simulink model "controla_planta_ROS"  (R2025b)
settings: Solver=ode14x  StartTime=0.0  StopTime=20  FixedStep=0.01  RelTol=1e-3
InitFcn:
  | start_time_epoch = posixtime(datetime('now'))-3600;
  | setenv('ROS_LOCALHOST_ONLY', '');
  | setenv('RMW_IMPLEMENTATION','rmw_cyclonedds_cpp')
values from neighbouring files (symbols this model uses):
  cc = 4.08    [parametros_planta.m]
  cp = 0.0002    [parametros_planta.m]
  g = 9.81    [parametros_planta.m]
  J = 0.0139    [parametros_planta.m]
  lcm = 0.3    [parametros_planta.m]
  M = mp + mc    (= 1.2)    [parametros_planta.m]
  mc = 1.08    [parametros_planta.m]
  mp = 0.12    [parametros_planta.m]
undefined symbols (not defined in the file or in its folder): K_lqr
libraries: ros2lib x2
settings Model: Creator=miguel  LastModifiedBy=miguel
settings SolverCC: EnableFixedStepZeroCrossing=on
settings OptimizationCC: DefaultParameterBehavior=Inlined  EnhancedBackFolding=on  PassReuseOutputArgsAs=Individual arguments  ZeroExternalMemoryAtStartup=off  ZeroInternalMemoryAtStartup=off  MaxStackSize=64  OptimizeBlockOrder=speed  DifferentSizesBufferReuse=on  OptimizationCustomize=off  EfficientTunableParamExpr=on
settings DebuggingCC: ParameterTunabilityLossMsg=error
settings HardwareCC: ProdBitPerLong=64.0  ProdHWDeviceType=Intel->x86-64 (Linux 64)  UseEmbeddedCoderFeatures=off
settings SFSimCC: MATLABDynamicMemAlloc=off
settings RTWCC: SystemTargetFile=ert.tlc  HardwareBoard=Robot Operating System 2 (ROS 2)  TLCOptions="-aInlineSetEventsForThisBaseRateFcn=TLC_FALSE -aSuppressMultiTaskScheduler=TLC_FALSE  -aRateBasedStepFcn=0"  TemplateMakefile=ert_default_tmf  Toolchain=Colcon Tools  TargetLang=C++  Description=Embedded Coder
settings CodeAppCC: ForceParamTrailComments=on  IgnoreCustomStorageClasses=off  OperatorAnnotations=on  SimulinkDataObjDesc=on  SFDataObjDesc=on  InsertBlockDesc=on
settings ERTTargetCC: ExtModeTransport=2.0  ExtModeStaticAlloc=on  ExtModeAutomaticAllocSize=off  ExtModeMexFile=ext_xcp  ExtModeIntrfLevel=Level2 - Open  RootIOFormat=Structure reference  CodeInterfacePackaging=C++ class  SupportNonInlinedSFcns=on

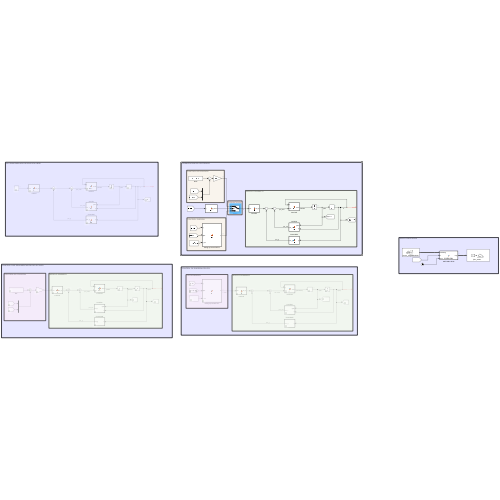
[thumbnail: Simulink's stored preview of the top-level diagram]
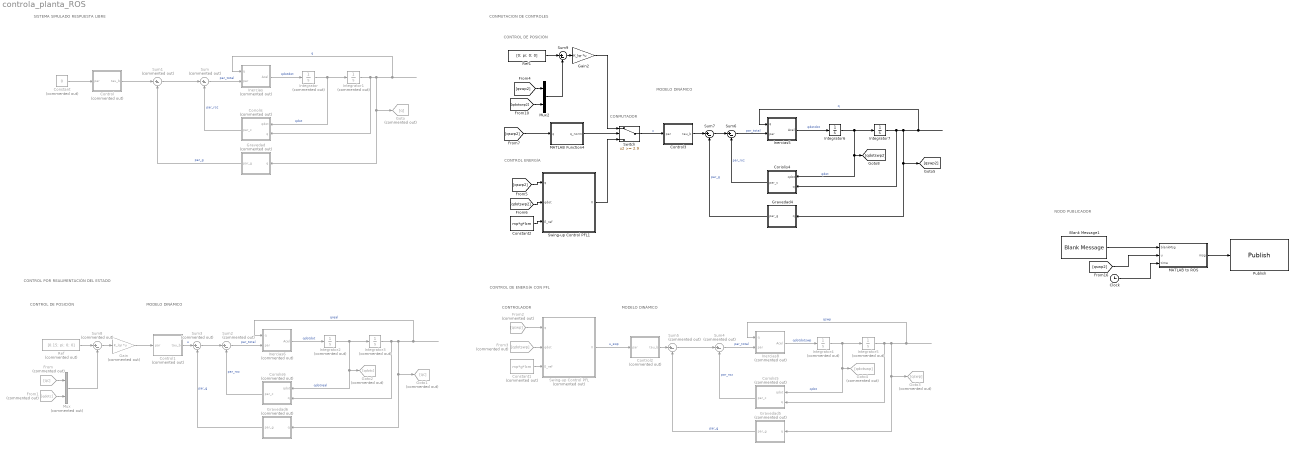
== system controla_planta_ROS ==
  note: CONTROLADOR
  note: MODELO DINÁMICO
  note: CONTROL DE POSICIÓN
  note: MODELO DINÁMICO
  note: CONMUTADOR
  note: MODELO DINÁMICO
  note: CONTROL ENERGÍA
  note: CONTROL DE POSICIÓN
  note: SISTEMA SIMULADO RESPUESTA LIBRE
  note: NODO PUBLICADOR
  note: CONTROL POR REALIMENTACIÓN DEL ESTADO
  note: CONTROL DE ENERGÍA CON PFL
  note: CONMUTACION DE CONTROLES
  Blank Message1 : ros2lib/Blank Message  messageClass=Message  entityType=sensor_msgs/JointState  messageType=sensor_msgs/JointState  SampleTime=inf
  Clock : Clock
  Constant : Constant  Commented=on  Value=0
  Constant1 : Constant  Commented=on  Value=mp*g*lcm
  Constant2 : Constant  Value=mp*g*lcm
  Control : MATLAB Function  Commented=on  TreatAsAtomicUnit=on
  Control1 : MATLAB Function  Commented=on  TreatAsAtomicUnit=on
  Control2 : MATLAB Function  Commented=on  TreatAsAtomicUnit=on
  Control3 : MATLAB Function  TreatAsAtomicUnit=on
  Coriolis : MATLAB Function  Commented=on  TreatAsAtomicUnit=on
  Coriolis4 : MATLAB Function  TreatAsAtomicUnit=on
  Coriolis5 : MATLAB Function  Commented=on  TreatAsAtomicUnit=on
  Coriolis6 : MATLAB Function  Commented=on  TreatAsAtomicUnit=on
  From : From  Commented=on  GotoTag=qc
  From1 : From  Commented=on  GotoTag=qdotc
  From2 : From  Commented=on  GotoTag=qswp
  From3 : From  Commented=on  GotoTag=qdotswp
  Gain : Gain  Commented=on  Gain=K_lqr  Multiplication=Matrix(K*u)
  Gain2 : Gain  Gain=K_lqr  Multiplication=Matrix(K*u)
  Goto : Goto  Commented=on  GotoTag=q
  Goto1 : Goto  Commented=on  GotoTag=qc
  Goto2 : Goto  Commented=on  GotoTag=qdotc
  Goto3 : Goto  Commented=on  GotoTag=qswp
  Goto4 : Goto  Commented=on  GotoTag=qdotswp
  Gravedad : MATLAB Function  Commented=on  TreatAsAtomicUnit=on
  Gravedad4 : MATLAB Function  TreatAsAtomicUnit=on
  Gravedad5 : MATLAB Function  Commented=on  TreatAsAtomicUnit=on
  Gravedad6 : MATLAB Function  Commented=on  TreatAsAtomicUnit=on
  Inercias : MATLAB Function  Commented=on  TreatAsAtomicUnit=on
  Inercias5 : MATLAB Function  TreatAsAtomicUnit=on
  Inercias6 : MATLAB Function  Commented=on  TreatAsAtomicUnit=on
  Inercias8 : MATLAB Function  Commented=on  TreatAsAtomicUnit=on
  Integrator : Integrator  Commented=on  InitialCondition=[0; 0]
  Integrator1 : Integrator  Commented=on  InitialCondition=[0; 3.14]
  Integrator2 : Integrator  Commented=on  InitialCondition=[0; 0]
  Integrator3 : Integrator  Commented=on  InitialCondition=[0; 3.20]
  Integrator4 : Integrator  Commented=on  InitialCondition=[0; 0.01]
  Integrator5 : Integrator  Commented=on  InitialCondition=[0; 0]
  Integrator6 : Integrator  InitialCondition=[0; 0.01]
  Integrator7 : Integrator  InitialCondition=[0; 0]
  MATLAB Function4 : MATLAB Function  TreatAsAtomicUnit=on
  MATLAB to ROS : MATLAB Function  TreatAsAtomicUnit=on
  Mux : Mux  Commented=on  Inputs=2
  Mux2 : Mux  Inputs=2
  Publish : ros2lib/Publish  topicSource=Specify your own  topic=/joint_states  messageType=sensor_msgs/JointState  QOSHistory=Keep last  QOSDepth=10  QOSReliability=Reliable  QOSDurability=Volatile  QOSDeadline=Inf  QOSLifespan=Inf  QOSLiveliness=Automatic  QOSLeaseDuration=Inf  QOSAvoidROSNamespaceConventions=off
  Ref : Constant  Commented=on  Value=[0.15; pi; 0; 0]
  Ref1 : Constant  Value=[0; pi; 0; 0]
  Sum{,1..5,8} (7 alike) : Sum  Commented=on  Inputs=|+-
  Sum6 : Sum  Inputs=|+-
  Sum7 : Sum  Inputs=|+-
  Sum9 : Sum  Inputs=|+-
  Swing-up Control PFL : MATLAB Function  Commented=on  TreatAsAtomicUnit=on
  Swing-up Control PFL1 : MATLAB Function  TreatAsAtomicUnit=on
  Switch : Switch  Threshold=2.9  SaturateOnIntegerOverflow=off  InputSameDT=off
  wires:
  Sum1/1 -> Sum/1
  Gravedad/1(par_g) -> Sum1/2  "par_g"
  Control/1(tau_b) -> Sum1/1
  Integrator1/1 -> Coriolis/2(q), Goto/1, Gravedad/1(q), Inercias/1(q)  "q"
  Inercias/1(Acel) -> Integrator/1  "qdotdot"
  Constant/1 -> Control/1(par)
  Integrator/1 -> Coriolis/1(qdot), Integrator1/1  "qdot"
  Sum/1 -> Inercias/2(par)  "par_total"
  Coriolis/1(par_c) -> Sum/2  "par_roz"
  Blank Message1/1 -> MATLAB to ROS/1(blankMsg)
  MATLAB to ROS/1(msg) -> Publish/1
  Clock/1 -> MATLAB to ROS/3(time)
  [qswp2] -> MATLAB to ROS/2(u)
  Coriolis6/1(par_c) -> Sum2/2  "par_roz"
  Control1/1(tau_b) -> Sum3/1  "u"
  Integrator3/1 -> Coriolis6/2(q), Gravedad6/1(q), Goto1/1, Inercias6/1(q)  "qreal"
  Inercias6/1(Acel) -> Integrator2/1  "qdotdot"
  Sum2/1 -> Inercias6/2(par)  "par_total"
  Gravedad6/1(par_g) -> Sum3/2  "par_g"
  Sum3/1 -> Sum2/1
  Integrator2/1 -> Coriolis6/1(qdot), Goto2/1, Integrator3/1  "qdotreal"
  From/1 -> Mux/1
  From1/1 -> Mux/2
  Inercias8/1(Acel) -> Integrator4/1  "qdotdotswp"
  Integrator5/1 -> Coriolis5/2(q), Gravedad5/1(q), Goto3/1, Inercias8/1(q)  "qswp"
  Sum5/1 -> Sum4/1
  Gravedad5/1(par_g) -> Sum5/2  "par_g"
  Control2/1(tau_b) -> Sum5/1
  Integrator4/1 -> Coriolis5/1(qdot), Goto4/1, Integrator5/1  "qdot"
  Sum4/1 -> Inercias8/2(par)  "par_total"
  Coriolis5/1(par_c) -> Sum4/2  "par_roz"
  Swing-up Control PFL/1(V) -> Control2/1(par)  "u_swp"
  From2/1 -> Swing-up Control PFL/1(q)
  From3/1 -> Swing-up Control PFL/2(qdot)
  Constant2/1 -> Swing-up Control PFL1/3(E_ref)
  Control3/1(tau_b) -> Sum7/1
  Coriolis4/1(par_c) -> Sum6/2  "par_roz"
  Sum7/1 -> Sum6/1
  Inercias5/1(Acel) -> Integrator6/1  "qdotdot"
  [qdotswp2] -> Swing-up Control PFL1/2(qdot)
  Integrator6/1 -> Coriolis4/1(qdot), [qdotswp2], Integrator7/1  "qdot"
  Sum6/1 -> Inercias5/2(par)  "par_total"
  [qswp2] -> Swing-up Control PFL1/1(q)
  Gravedad4/1(par_g) -> Sum7/2  "par_g"
  Integrator7/1 -> Coriolis4/2(q), Gravedad4/1(q), [qswp2], Inercias5/1(q)  "q"
  Switch/1 -> Control3/1(par)  "u"
  MATLAB Function4/1(q_norm) -> Switch/2
  [qswp2] -> MATLAB Function4/1(q)
  Constant1/1 -> Swing-up Control PFL/3(E_ref)
  Mux/1 -> Sum8/2
  Ref/1 -> Sum8/1
  Gain/1 -> Control1/1(par)
  Sum8/1 -> Gain/1
  Ref1/1 -> Sum9/1
  [qswp2] -> Mux2/1
  Mux2/1 -> Sum9/2
  Sum9/1 -> Gain2/1
  [qdotswp2] -> Mux2/2
  Swing-up Control PFL1/1(V) -> Switch/3
  Gain2/1 -> Switch/1

== matlab function controla_planta_ROS/Control2 ==
  data: par input; tau_b output
function tau_b = B(par)

tau_b = [0.64; 0]*par; %Nuestra acción de control se aplica sobre el eje horizontal.

== matlab function controla_planta_ROS/Gravedad5 ==
  data: q input; par_g output; mp parameter; g parameter; lcm parameter
function par_g = Gq(q, mp, g, lcm)
G = [0; mp*g*lcm*sin(q(2))]; 

par_g = G;

== matlab function controla_planta_ROS/Coriolis5 ==
  data: qdot input; q input; par_c output size=[2, 1]; cc parameter; cp parameter; mp parameter; lcm parameter
function par_c = Cq(qdot, q, cc, cp, mp, lcm)

%Nota: cp = 0 Nm.rad/s no me lo creo habrá que estimarlo de forma
%conservadora.

C = [cc,   -mp*lcm*qdot(2)*sin(q(2))
      0,          cp        ]; 

par_c = C*qdot;

== matlab function controla_planta_ROS/Control3 ==
  data: par input; tau_b output
function tau_b = B(par)

tau_b = [0.64; 0]*par; %Nuestra acción de control se aplica sobre el eje horizontal.

== matlab function controla_planta_ROS/Swing-up Control PFL ==
  data: q input; V output; qdot input; E_ref input; mp parameter; lcm parameter; cp parameter; cc parameter; J parameter; mc parameter
function V = fcn(q, qdot, E_ref, mp, lcm, cp, cc, J, mc) % Añadido Mc y salida F

% --- PARAMETROS FISICOS Y GANANCIAS ---
g = 9.81; % Añadido el punto y coma

% Ganancias del control de energía (Swing-up) AJUSTAR
Ke = 50; 
kp = 8.16; 
kd = 4; 

% -- ESTADOS DEL SISTEMA --
x = q(1);        % Posición del carro
theta = q(2);    % Ángulo del péndulo (0 = arriba)
xdot = qdot(1);  % Velocidad del carro
thetadot = qdot(2); % Velocidad angular

% --- 1. CÁLCULO DE ENERGÍA ---
Ep = -mp * g * lcm * cos(theta); 
Ek = 0.5 * J * thetadot^2;
E_total = Ep + Ek;

% --- 2. LEY DE CONTROL DE ENERGÍA (Aceleración 'u') ---
e = E_total - E_ref;
u = Ke * thetadot * cos(theta) * e - kp * x - kd * xdot;

% --- 3. LINEARIZACIÓN POR RETROALIMENTACIÓN PARCIAL (PFL) ---
% Convierte la aceleración deseada 'u' en Fuerza 'F' para el motor

thetadotdot = 1/J *(-mp*lcm*cos(theta)*u ...
    + mp*g*lcm*sin(theta) -cp*thetadot);

F = (mc + mp) * u ...
    - (mp * lcm * thetadot^2 * sin(theta)) ...
    + (mp * lcm * cos(theta)) * thetadotdot ...
    +cc*xdot;

%Saturacion --> Evitar oscilaciones iniciales bruscas.
F_max = 4; % Newtons
if F > F_max
    F = F_max;
elseif F < -F_max
    F = -F_max;
end

V = F / 0.64;   %Conversión a voltios

end

== matlab function controla_planta_ROS/Gravedad6 ==
  data: q input; par_g output; mp parameter; g parameter; lcm parameter
function par_g = Gq(q, mp, g, lcm)
G = [0; mp*g*lcm*sin(q(2))]; 

par_g = G;

== matlab function controla_planta_ROS/Coriolis6 ==
  data: qdot input; q input; par_c output size=[2, 1]; cc parameter; cp parameter; mp parameter; lcm parameter
function par_c = Cq(qdot, q, cc, cp, mp, lcm)

%Nota: cp = 0 Nm.rad/s no me lo creo habrá que estimarlo de forma
%conservadora.

C = [cc,   -mp*lcm*qdot(2)*sin(q(2))
      0,          cp        ]; 

par_c = C*qdot;

== matlab function controla_planta_ROS/MATLAB Function4 ==
  data: q input; q_norm output
function q_norm = fcn(q)
    % Esto envuelve el ángulo para que siempre esté entre -pi y +pi
    q_norm = atan2(sin(q(2)), cos(q(2)));
    q_norm = abs(q_norm);
end

== matlab function controla_planta_ROS/MATLAB to ROS ==
  data: blankMsg input; msg output Bus: SL_Bus_sensor_msgs_JointState; u input; time input; start_time_epoch parameter
function msg = create_msg(blankMsg, u, time, start_time_epoch)
%#codegen
msg = blankMsg;

%Sincronización con el reloj interno de la máquina.
total_time = start_time_epoch + time; 
%Indicar el tiempo de simulación para que RViz pueda componer la
%simulación. 
s = floor(total_time);
ns = (total_time - s) * 1e9;  
msg.header.stamp.sec = int32(s);
msg.header.stamp.nanosec = uint32(ns);

% Definimos los nombres y sus posiciones correspondientes
strArrayToAssign = {'cart_slider', 'pole_joint'};
% Las posiciones angulares de nuestro péndulo. 
positionsToAssign = [u(1), u(2)]; 

% 1. Configurar NOMBRES (Strings)
numStringsInArray = length(strArrayToAssign);
msg.name_SL_Info.CurrentLength = uint32(numStringsInArray);

for idx=1:numStringsInArray
    str = strArrayToAssign{idx};
    strLength = length(str);
    % Asignar caracteres convertidos a uint8
    msg.name(idx).data(1:strLength) = uint8(str);
    msg.name(idx).data_SL_Info.CurrentLength = uint32(strLength);
end

% 2. Configurar POSICIONES (float64 array)
% El campo 'position' en un Bus de Simulink para JointState 
% también tiene un campo _SL_Info asociado para controlar la longitud.
numPositions = length(positionsToAssign);
msg.position_SL_Info.CurrentLength = uint32(numPositions);
% Asignamos los valores directamente
msg.position(1:numPositions) = positionsToAssign;

% 3. Dejar sin campo de velocidad y esfuerzo el tópico.
msg.velocity_SL_Info.CurrentLength = uint32(0);
msg.effort_SL_Info.CurrentLength = uint32(0);

end

== matlab function controla_planta_ROS/Inercias5 ==
  data: q input; par input; Acel output; J parameter; M parameter; mp parameter; lcm parameter
function Acel = Minv(q,par, J, M, mp, lcm)
%La matriz va aumentando su dimensionalidad a medida que se añaden GDLs

M = [M,          +mp*lcm*cos(q(2));
    +mp*lcm*cos(q(2)),      J]; 

Acel = M\par; %División de matrices.

== matlab function controla_planta_ROS/Coriolis ==
  data: qdot input; q input; par_c output size=[2, 1]; cc parameter; cp parameter; mp parameter; lcm parameter
function par_c = Cq(qdot, q, cc, cp, mp, lcm)

%Nota: cp = 0 Nm.rad/s no me lo creo habrá que estimarlo de forma
%conservadora.

C = [cc,   -mp*lcm*qdot(2)*sin(q(2))
      0,          cp        ]; 

par_c = C*qdot;

== matlab function controla_planta_ROS/Inercias6 ==
  data: q input; par input; Acel output; J parameter; M parameter; mp parameter; lcm parameter
function Acel = Minv(q,par, J, M, mp, lcm)
%La matriz va aumentando su dimensionalidad a medida que se añaden GDLs

M = [M,          +mp*lcm*cos(q(2));
    +mp*lcm*cos(q(2)),      J]; 

Acel = M\par; %División de matrices.

== matlab function controla_planta_ROS/Inercias8 ==
  data: q input; par input; Acel output; J parameter; M parameter; mp parameter; lcm parameter
function Acel = Minv(q,par, J, M, mp, lcm)
%La matriz va aumentando su dimensionalidad a medida que se añaden GDLs

M = [M,          +mp*lcm*cos(q(2));
    +mp*lcm*cos(q(2)),      J]; 

Acel = M\par; %División de matrices.

== matlab function controla_planta_ROS/Inercias ==
  data: q input; par input; Acel output; J parameter; M parameter; mp parameter; lcm parameter
function Acel = Minv(q,par, J, M, mp, lcm)
%La matriz va aumentando su dimensionalidad a medida que se añaden GDLs

M = [M,          +mp*lcm*cos(q(2));
    +mp*lcm*cos(q(2)),      J]; 

Acel = M\par; %División de matrices.

== matlab function controla_planta_ROS/Gravedad ==
  data: q input; par_g output; mp parameter; g parameter; lcm parameter
function par_g = Gq(q, mp, g, lcm)
G = [0; mp*g*lcm*sin(q(2))]; 

par_g = G;

== matlab function controla_planta_ROS/Control ==
  data: par input; tau_b output
function tau_b = B(par)

tau_b = [0.64; 0]*par; %Nuestra acción de control se aplica sobre el eje horizontal.

== matlab function controla_planta_ROS/Control1 ==
  data: par input; tau_b output
function tau_b = B(par)

tau_b = [0.64; 0]*par; %Nuestra acción de control se aplica sobre el eje horizontal.

== matlab function controla_planta_ROS/Gravedad4 ==
  data: q input; par_g output; mp parameter; g parameter; lcm parameter
function par_g = Gq(q, mp, g, lcm)
G = [0; mp*g*lcm*sin(q(2))]; 

par_g = G;

== matlab function controla_planta_ROS/Swing-up Control PFL1 ==
  data: q input; V output; qdot input; E_ref input; mp parameter; lcm parameter; cp parameter; cc parameter; J parameter; mc parameter
function V = fcn(q, qdot, E_ref, mp, lcm, cp, cc, J, mc) % Añadido Mc y salida F

% --- PARAMETROS FISICOS Y GANANCIAS ---
g = 9.81; % Añadido el punto y coma

% Ganancias del control de energía (Swing-up) AJUSTAR
Ke = 50; 
kp = 8.16; 
kd = 4; 

% -- ESTADOS DEL SISTEMA --
x = q(1);        % Posición del carro
theta = q(2);    % Ángulo del péndulo (0 = arriba)
xdot = qdot(1);  % Velocidad del carro
thetadot = qdot(2); % Velocidad angular

% --- 1. CÁLCULO DE ENERGÍA ---
Ep = -mp * g * lcm * cos(theta); 
Ek = 0.5 * J * thetadot^2;
E_total = Ep + Ek;

% --- 2. LEY DE CONTROL DE ENERGÍA (Aceleración 'u') ---
e = E_total - E_ref;
u = Ke * thetadot * cos(theta) * e - kp * x - kd * xdot;

% --- 3. LINEARIZACIÓN POR RETROALIMENTACIÓN PARCIAL (PFL) ---
% Convierte la aceleración deseada 'u' en Fuerza 'F' para el motor

thetadotdot = 1/J *(-mp*lcm*cos(theta)*u ...
    + mp*g*lcm*sin(theta) -cp*thetadot);

F = (mc + mp) * u ...
    - (mp * lcm * thetadot^2 * sin(theta)) ...
    + (mp * lcm * cos(theta)) * thetadotdot ...
    +cc*xdot;

%Saturacion --> Evitar oscilaciones iniciales bruscas.
F_max = 4; % Newtons
if F > F_max
    F = F_max;
elseif F < -F_max
    F = -F_max;
end

V = F / 0.64;   %Conversión a voltios

end

== matlab function controla_planta_ROS/Coriolis4 ==
  data: qdot input; q input; par_c output size=[2, 1]; cc parameter; cp parameter; mp parameter; lcm parameter
function par_c = Cq(qdot, q, cc, cp, mp, lcm)

%Nota: cp = 0 Nm.rad/s no me lo creo habrá que estimarlo de forma
%conservadora.

C = [cc,   -mp*lcm*qdot(2)*sin(q(2))
      0,          cp        ]; 

par_c = C*qdot;
